simulink model "lookup_nD_TestGen12"  (R2017b)
settings: Solver=FixedStepDiscrete  StartTime=0.0  StopTime=10.0  RelTol=1e-3
model workspace (MAT data in the model file):
  LUTObjLKnD12 = Simulink.LookupTable
  LUTObjLKnD12.Table = Simulink.lookuptable.Table
  LUTObjLKnD12.Table.Value = [104.545305439  12.3883152177  56.0568425054  110.028262146  33.0224434571; 20.8267841797  97.8066958134  16.5897343715  8.34661927516  56.7644043811; 26.1209276873  125.059269707  31.1150866489  7.66307185203  85.7450031938]
  LUTObjLKnD12.Table.Dimensions = [3 5]
  LUTObjLKnD12.Table.DataType = 'auto'
  LUTObjLKnD12.Table.FieldName = 'Table'
  LUTObjLKnD12.BreakpointsSpecification = 'Even spacing'
  LUTObjLKnD12.Breakpoints(1) = Simulink.lookuptable.Evenspacing
  LUTObjLKnD12.Breakpoints(1).FirstPoint = 33.2086127016
  LUTObjLKnD12.Breakpoints(1).Spacing = 1.5
  LUTObjLKnD12.Breakpoints(1).FirstPointName = 'BPFirstPoint1'
  LUTObjLKnD12.Breakpoints(1).SpacingName = 'BPSpacing1'
  LUTObjLKnD12.Breakpoints(1).TunableSizeName = 'N1'
  LUTObjLKnD12.Breakpoints(1).DataType = 'auto'
  LUTObjLKnD12.Breakpoints(1).FieldName = 'BP1'
  LUTObjLKnD12.Breakpoints(2) = Simulink.lookuptable.Evenspacing
  LUTObjLKnD12.Breakpoints(2).FirstPoint = 88.4144489995
  LUTObjLKnD12.Breakpoints(2).Spacing = 1.5
  LUTObjLKnD12.Breakpoints(2).FirstPointName = 'BPFirstPoint2'
  LUTObjLKnD12.Breakpoints(2).SpacingName = 'BPSpacing2'
  LUTObjLKnD12.Breakpoints(2).TunableSizeName = 'N2'
  LUTObjLKnD12.Breakpoints(2).DataType = 'auto'
  LUTObjLKnD12.Breakpoints(2).FieldName = 'BP2'
  LUTObjLKnD12.SupportTunableSize = 0
  LUTObjLKnD12.StructTypeInfo = Simulink.lookuptable.StructTypeInfo
  LUTObjLKnD12.StructTypeInfo.Name = 'LUT'
  LUTObjLKnD12.StructTypeInfo.DataScope = 'Auto'
settings Model: Creator=ktrinh  LastModifiedBy=ktrinh
settings DebuggingCC: ParameterOverflowMsg=none

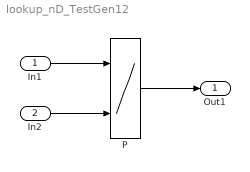
== system lookup_nD_TestGen12 ==
  In1 : Inport  OutMin=0  OutMax=127  PortDimensions=3
  In2 : Inport  Port=2  OutMin=0  OutMax=127
  P : Lookup_n-D  DataSpecification=Lookup table object  LookupTableObject=LUTObjLKnD12  BreakpointsSpecification=Even spacing  BreakpointsForDimension3=[5, 7]  Table=reshape(repmat([4 5 6;16 19 20;10 18 23],1,2),[3,3,2])  UseLastTableValue=on  InternalRulePriority=Speed  RndMeth=Simplest  InputSameDT=on
  Out1 : Outport
  wires:
  In1/1 -> P/1
  In2/1 -> P/2
  P/1 -> Out1/1
